simulink model "Ziegler"  (Simulink 5.0)
settings: Solver=ode4  StartTime=0.0  StopTime=15  FixedStep=0.25  RelTol=1e-3
values from neighbouring files (symbols this model uses):
  kd = kp*pi/(4*wr)    [ZieglerDm4_29.m]    (also in Zieglerm4_27.m; example4_15.m = 0.01; example4_16.m = 0.006)
  ki = kp*wr/pi    [ZieglerDm4_29.m]    (also in Zieglerm4_27.m; example4_15.m = 1; example4_16.m = 0.01)
  kp = 0.6*kr    [ZieglerDm4_29.m]    (also in Zieglerm4_27.m; example4_15.m = 1.5; example4_16.m = 1.9)
libraries: simulink x3
settings Model: LastModifiedBy=Administrator  ExtModeTrigMode=oneshot  ExtModeArmWhenConnect=off  LimitDataPoints=off  BooleanDataType=off

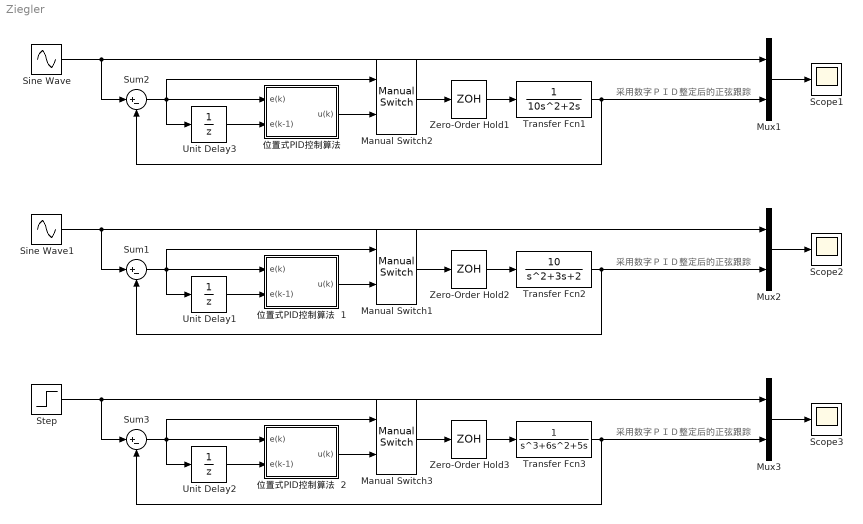
== system Ziegler ==
  note: 采用数字ＰＩＤ整定后的正弦跟踪
  note: 采用数字ＰＩＤ整定后的正弦跟踪
  note: 采用数字ＰＩＤ整定后的正弦跟踪
  Manual Switch1 : simulink/Signal Routing/Manual Switch  sw=1  action=0
  Manual Switch2 : simulink/Signal Routing/Manual Switch  sw=0  action=0
  Manual Switch3 : simulink/Signal Routing/Manual Switch  sw=0  action=0
  Mux1 : Mux  Inputs=2
  Mux2 : Mux  Inputs=2
  Mux3 : Mux  Inputs=2
  Scope1 : Scope
      settings: YMin=-3.5  YMax=1  MaxDataPoints=500000
  Scope2 : Scope
      settings: YMin=-3.5  YMax=1  MaxDataPoints=500000
  Scope3 : Scope
      settings: YMin=-3.5  YMax=1  SaveName=ScopeData2  MaxDataPoints=500000
  Sine Wave : Sin  Amplitude=0.5  Frequency=0.05*pi  SampleTime=0
  Sine Wave1 : Sin  Amplitude=0.5  Frequency=0.05*pi  SampleTime=0
  Step : Step  SampleTime=0
  Sum1 : Sum  Inputs=|+-  SaturateOnIntegerOverflow=on
  Sum2 : Sum  Inputs=|+-  SaturateOnIntegerOverflow=on
  Sum3 : Sum  Inputs=|+-  SaturateOnIntegerOverflow=on
  Transfer Fcn1 : TransferFcn  Denominator=[10,2,0]
  Transfer Fcn2 : TransferFcn  Numerator=[10]  Denominator=[1,3,2]
  Transfer Fcn3 : TransferFcn  Denominator=[1,6,5 0]
  Unit Delay1 : UnitDelay  SampleTime=0.25
  Unit Delay2 : UnitDelay  SampleTime=0.25
  Unit Delay3 : UnitDelay  SampleTime=0.25
  Zero-Order Hold1 : ZeroOrderHold  SampleTime=0.25
  Zero-Order Hold2 : ZeroOrderHold  SampleTime=0.25
  Zero-Order Hold3 : ZeroOrderHold  SampleTime=0.25
  "位置式PID控制算法  " : Subsystem
  位置式PID控制算法  1 : Subsystem
  位置式PID控制算法  2 : Subsystem
  wires:
  Sine Wave/1 -> Sum2/1, Mux1/1
  Mux1/1 -> Scope1/1
  Transfer Fcn1/1 -> Sum2/2, Mux1/2
  Unit Delay3/1 -> "位置式PID控制算法  "/2(e(k-1))
  Sum2/1 -> "位置式PID控制算法  "/1(e(k)), Manual Switch2/1, Unit Delay3/1
  "位置式PID控制算法  "/1(u(k)) -> Manual Switch2/2
  Zero-Order Hold1/1 -> Transfer Fcn1/1
  Manual Switch2/1 -> Zero-Order Hold1/1
  Sine Wave1/1 -> Mux2/1, Sum1/1
  Mux2/1 -> Scope2/1
  Transfer Fcn2/1 -> Mux2/2, Sum1/2
  Unit Delay1/1 -> 位置式PID控制算法  1/2(e(k-1))
  Sum1/1 -> Unit Delay1/1, Manual Switch1/1, 位置式PID控制算法  1/1(e(k))
  位置式PID控制算法  1/1(u(k)) -> Manual Switch1/2
  Zero-Order Hold2/1 -> Transfer Fcn2/1
  Manual Switch1/1 -> Zero-Order Hold2/1
  Step/1 -> Sum3/1, Mux3/1
  Mux3/1 -> Scope3/1
  Transfer Fcn3/1 -> Sum3/2, Mux3/2
  Unit Delay2/1 -> 位置式PID控制算法  2/2(e(k-1))
  Sum3/1 -> 位置式PID控制算法  2/1(e(k)), Manual Switch3/1, Unit Delay2/1
  位置式PID控制算法  2/1(u(k)) -> Manual Switch3/2
  Zero-Order Hold3/1 -> Transfer Fcn3/1
  Manual Switch3/1 -> Zero-Order Hold3/1

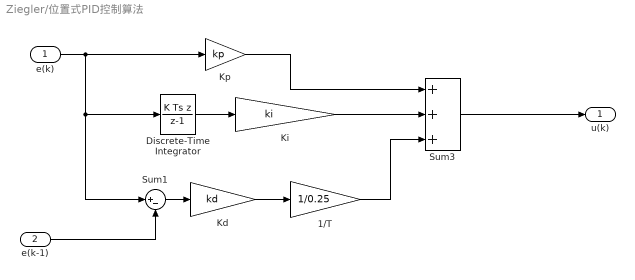
== system Ziegler/位置式PID控制算法   ==
  e(k) : Inport
  e(k-1) : Inport  Port=2
  1/T : Gain  Gain=1/0.25  SaturateOnIntegerOverflow=on
  Discrete-Time Integrator : DiscreteIntegrator  IntegratorMethod=Backward Euler  SampleTime=0.25
  Kd : Gain  Gain=kd  SaturateOnIntegerOverflow=on
  Ki : Gain  Gain=ki  SaturateOnIntegerOverflow=on
  Kp : Gain  Gain=kp  SaturateOnIntegerOverflow=on
  Sum1 : Sum  Inputs=|+-  SaturateOnIntegerOverflow=on
  Sum3 : Sum  Inputs=+++  SaturateOnIntegerOverflow=on
  u(k) : Outport
  wires:
  e(k-1)/1 -> Sum1/2
  1/T/1 -> Sum3/3
  Kd/1 -> 1/T/1
  Sum3/1 -> u(k)/1
  Ki/1 -> Sum3/2
  Kp/1 -> Sum3/1
  e(k)/1 -> Sum1/1, Discrete-Time Integrator/1, Kp/1
  Sum1/1 -> Kd/1
  Discrete-Time Integrator/1 -> Ki/1

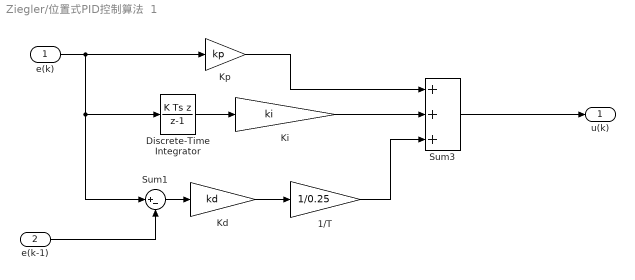
== system Ziegler/位置式PID控制算法  1 ==
  e(k) : Inport
  e(k-1) : Inport  Port=2
  1/T : Gain  Gain=1/0.25  SaturateOnIntegerOverflow=on
  Discrete-Time Integrator : DiscreteIntegrator  IntegratorMethod=Backward Euler  SampleTime=0.25
  Kd : Gain  Gain=kd  SaturateOnIntegerOverflow=on
  Ki : Gain  Gain=ki  SaturateOnIntegerOverflow=on
  Kp : Gain  Gain=kp  SaturateOnIntegerOverflow=on
  Sum1 : Sum  Inputs=|+-  SaturateOnIntegerOverflow=on
  Sum3 : Sum  Inputs=+++  SaturateOnIntegerOverflow=on
  u(k) : Outport
  wires:
  Discrete-Time Integrator/1 -> Ki/1
  Sum1/1 -> Kd/1
  e(k)/1 -> Kp/1, Discrete-Time Integrator/1, Sum1/1
  Kp/1 -> Sum3/1
  Ki/1 -> Sum3/2
  Sum3/1 -> u(k)/1
  Kd/1 -> 1/T/1
  1/T/1 -> Sum3/3
  e(k-1)/1 -> Sum1/2

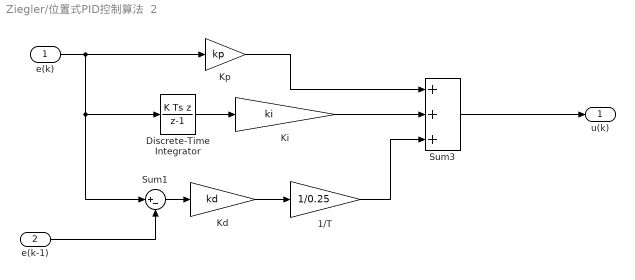
== system Ziegler/位置式PID控制算法  2 ==
  e(k) : Inport
  e(k-1) : Inport  Port=2
  1/T : Gain  Gain=1/0.25  SaturateOnIntegerOverflow=on
  Discrete-Time Integrator : DiscreteIntegrator  IntegratorMethod=Backward Euler  SampleTime=0.25
  Kd : Gain  Gain=kd  SaturateOnIntegerOverflow=on
  Ki : Gain  Gain=ki  SaturateOnIntegerOverflow=on
  Kp : Gain  Gain=kp  SaturateOnIntegerOverflow=on
  Sum1 : Sum  Inputs=|+-  SaturateOnIntegerOverflow=on
  Sum3 : Sum  Inputs=+++  SaturateOnIntegerOverflow=on
  u(k) : Outport
  wires:
  e(k-1)/1 -> Sum1/2
  1/T/1 -> Sum3/3
  Kd/1 -> 1/T/1
  Sum3/1 -> u(k)/1
  Ki/1 -> Sum3/2
  Kp/1 -> Sum3/1
  e(k)/1 -> Sum1/1, Discrete-Time Integrator/1, Kp/1
  Sum1/1 -> Kd/1
  Discrete-Time Integrator/1 -> Ki/1
